simulink model "QuadEncoder_SFunction_carion"  (R2013a)
settings: Solver=FixedStepDiscrete  SolverMode=SingleTasking  StartTime=0.0  StopTime=inf  FixedStep=35e-3  RelTol=1e-3
settings Model: SimulationMode=external  ExtModeTrigDuration=2  Creator=Alec  LastModifiedBy=carion10
settings OptimizationCC: ExpressionDepthLimit=2147483647  OptimizeModelRefInitCode=on  LifeSpan=1
settings DebuggingCC: SolverPrmCheckMsg=none  StrictBusMsg=Warning
settings HardwareCC: ProdBitPerInt=16  ProdBitPerPointer=8  ProdIntDivRoundTo=Zero  ProdEndianess=LittleEndian  ProdWordSize=8  ProdHWDeviceType=Atmel->AVR
settings RTWCC: SystemTargetFile=realtime.tlc  GenerateMakefile=off  TemplateMakefile=realtime.tmf  Description=Real-Time Toolbox  RTWVerbose=off  ProcessScript=realtime_make_rtw_hook
settings CodeAppCC: CustomSymbolStrType=$N$R$M  InternalIdentifier=Classic
settings STFCustomTargetCC: TargetLibSuffix=.a  GenerateSampleERTMain=on  ERTCustomFileBanners=on  SupportNonInlinedSFcns=off  SupportVariableSizeSignals=on  MATLABClassNameForMDSCustomization=Simulink.SoftwareTarget.ERTCustomization  SystemTargetFile=realtime.tlc
settings ERTTargetCC: ParMdlRefBuildCompliant=off  CompOptLevelCompliant=off  ConcurrentExecutionCompliant=off  CombineOutputUpdateFcns=off  ERTFirstTimeCompliant=off  SupportContinuousTime=on  SupportVariableSizeSignals=on  ModelStepFunctionPrototypeControlCompliant=off  CPPClassGenCompliant=off  ExtMode=on  ExtModeTransport=3  ExtModeMexFile=ext_serial_win32_comm  ExtModeMexArgs=0 7 115200  ERTSrcFileBannerTemplate=realtime_code_template.cgt  ERTHdrFileBannerTemplate=realtime_code_template.cgt  ERTDataSrcFileTemplate=realtime_code_template.cgt  ERTDataHdrFileTemplate=realtime_code_template.cgt  ERTCustomFileTemplate=realtime_file_process.tlc

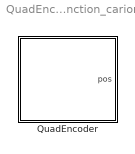
== system QuadEncoder_SFunction_carion ==
  QuadEncoder : Subsystem

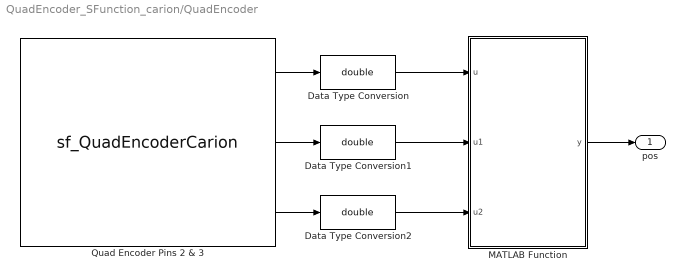
== system QuadEncoder_SFunction_carion/QuadEncoder ==
  Data Type Conversion : DataTypeConversion  OutDataTypeStr=double
  Data Type Conversion1 : DataTypeConversion  OutDataTypeStr=double
  Data Type Conversion2 : DataTypeConversion  OutDataTypeStr=double
  MATLAB Function : MATLAB Function  TreatAsAtomicUnit=on
  Quad Encoder Pins 2 & 3 : S-Function  InitFcn=try, set_param(gcb,'FunctionName','sf_QuadEncoderCarion'), end  FunctionName=sf_QuadEncoderCarion  Parameters=uint8(0),uint8(2),uint8(3)  SFunctionModules=sf_QuadEncoderCarion_wrapper  EnableBusSupport=off  mask(S-Function Builder){}
      mask init:
      | val = [[.9  0.75 0.75 1 1 .9 .9 1]',[1 1 0.75 0.75 .9 .9 1 .9]'];try , sys = get_param(gcb,'SfunBuilderFcnName');if isempty(sys), sys = get_param(gcb,'FunctionName'); end,catch, sys = get_param(gcb,'FunctionName'); end
      settings: CopyFcn=set_param(gcbh,'LinkStatus','none')  PreSaveFcn=try, set_param(gcb,'FunctionName','sf_QuadEncoderCarion'), end  OpenFcn=sfunctionwizard(gcbh)
      mask Display: plot(val(:,1),val(:,2)),disp(sys), port_label('output',1,'pos'), port_label('output',2,'overflow'), port_label('output',3,'underflow')
  pos : Outport
  wires:
  Data Type Conversion/1 -> MATLAB Function/1(u)
  Data Type Conversion1/1 -> MATLAB Function/2(u1)
  Data Type Conversion2/1 -> MATLAB Function/3(u2)
  Quad Encoder Pins 2 & 3/1 -> Data Type Conversion/1
  MATLAB Function/1(y) -> pos/1
  Quad Encoder Pins 2 & 3/2 -> Data Type Conversion1/1
  Quad Encoder Pins 2 & 3/3 -> Data Type Conversion2/1

== matlab function QuadEncoder_SFunction_carion/QuadEncoder/MATLAB Function ==
  data: u input; y output; u1 input; u2 input
function y = fcn(u,u1,u2)
%#codegen
max = 32767;
min = -32767;

y = u1*max + u2*min + u;
